simulink model "ExampleMotive_control_comnmunication"  (R2015a)
settings: Solver=ode1  StartTime=0.0  StopTime=inf  FixedStep=0.2  RelTol=1e-3
InitFcn:
  | fig_h = figure;
  | ax_h = axes;
  | set(ax_h,'Xlim',[-100 100],'YLim',[-100 100])
settings Model: ExtModeTrigDuration=5000  Creator=adm-drone  LastModifiedBy=jitesh_esb201
settings SolverCC: PositivePriorityOrder=on
settings DebuggingCC: UnderspecifiedInitializationDetection=Classic  MergeDetectMultiDrivingBlocksExec=none  SolverPrmCheckMsg=warning  StateNameClashWarn=warning
settings RTWCC: SystemTargetFile=quarc_win64.tlc  TemplateMakefile=quarc_default_tmf  Description=QUARC Win64 Target
settings STFCustomTargetCC: TargetLibSuffix=.lib  TargetPreCompLibLocation=C:\PROGRA~3\QUARC\lib\2013a\win64\release  GenerateSampleERTMain=off  GeneratePreprocessorConditionals=Disable all  CombineOutputUpdateFcns=on  ERTCustomFileBanners=off  SupportNonInlinedSFcns=on  SupportVariableSizeSignals=off  MATLABClassNameForMDSCustomization=Simulink.SoftwareTarget.GRTCustomization  CPPClassGenCompliant=on  SystemTargetFile=quarc_win64.tlc
settings GRTTargetCC: TargetPreCompLibLocation=C:\PROGRA~3\QUARC\lib\2013a\win64\release  ParMdlRefBuildCompliant=off  CompOptLevelCompliant=off  ConcurrentExecutionCompliant=off  MatFileLogging=off  ExtMode=on  ExtModeMexFile=quarc_comm

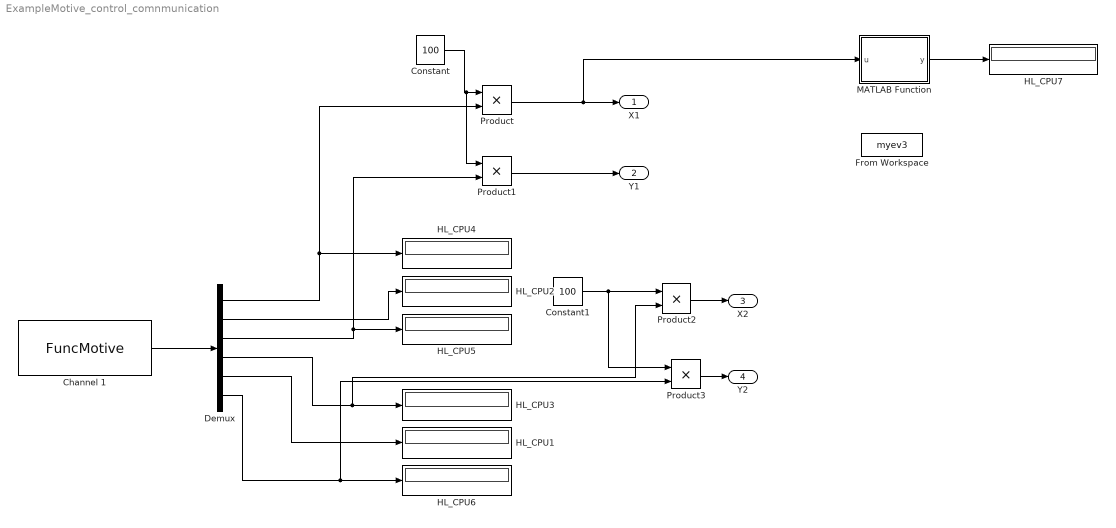
== system ExampleMotive_control_comnmunication ==
  Channel 1 : M-S-Function  FunctionName=FuncMotive  Parameters=1
  Constant : Constant  Value=100
  Constant1 : Constant  Value=100
  Demux : Demux  Outputs=6
  From Workspace : FromWorkspace  VariableName=myev3  SampleTime=0
  HL_CPU{1..7} (7 alike) : Display
  MATLAB Function : MATLAB Function  TreatAsAtomicUnit=on
  Product{,1..3} (4 alike) : Product
  X1 : Outport
  Y1 : Outport  Port=2
  X2 : Outport  Port=3
  Y2 : Outport  Port=4
  wires:
  Channel 1/1 -> Demux/1
  Demux/1 -> Product/2, HL_CPU4/1
  Demux/2 -> HL_CPU2/1
  Demux/3 -> HL_CPU5/1, Product1/2
  Constant/1 -> Product1/1, Product/1
  Demux/4 -> Product2/2, HL_CPU3/1
  Demux/5 -> HL_CPU1/1
  Demux/6 -> Product3/2, HL_CPU6/1
  Product/1 -> MATLAB Function/1(u), X1/1
  Product1/1 -> Y1/1
  Constant1/1 -> Product3/1, Product2/1
  Product2/1 -> X2/1
  Product3/1 -> Y2/1
  MATLAB Function/1(y) -> HL_CPU7/1

== matlab function ExampleMotive_control_comnmunication/MATLAB Function ==
  data: u input; y output
function y = fcn(u)
%#codegen
mymotor_A = motor(myev3,'A');
mymotor_B = motor(myev3,'B')

mymotor_A.Speed = -50;
mymotor_B.Speed = -20;
start(mymotor_A)
start(mymotor_B)
pause(10)
stop(mymotor_A)
stop(mymotor_B)
y = u;
